simulink model "feedback_harness"  (R2013a)
settings: Solver=ode45  StartTime=0.0  StopTime=8  RelTol=1e-3
settings Model: ModifiedByFormat=The MathWorks Inc.  Creator=The MathWorks Inc.  LastModifiedBy=The MathWorks Inc.
settings DataIOCC: SaveOutput=off  SaveTime=off
settings OptimizationCC: ExpressionDepthLimit=2147483647  LifeSpan=1
settings DebuggingCC: FcnCallInpInsideContextMsg=EnableAllAsWarning
settings GRTTargetCC: CombineOutputUpdateFcns=off  GRTInterface=on

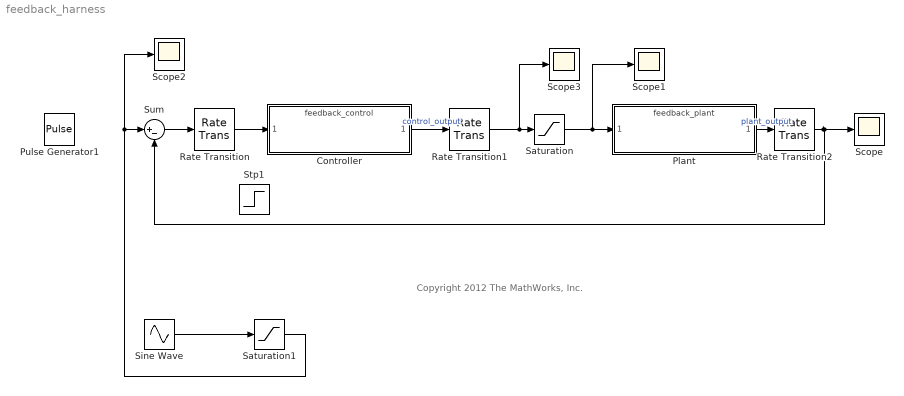
== system feedback_harness ==
  note: Copyright 2012 The MathWorks, Inc.
  Controller : ModelReference  ModelNameDialog=feedback_control  SimulationMode=Normal  ModelReferenceVersion=1.59  CopyOfModelName=feedback_control  DefaultDataLogging=on
  Plant : ModelReference  ModelNameDialog=feedback_plant  SimulationMode=Normal  ModelReferenceVersion=1.26  CopyOfModelName=feedback_plant  DefaultDataLogging=on
  Pulse Generator1 : DiscretePulseGenerator  Period=4000  PulseWidth=2000  SampleTime=0.001
  Rate Transition : RateTransition
  Rate Transition1 : RateTransition  OutPortSampleTime=0.001
  Rate Transition2 : RateTransition
  Saturation : Saturate  UpperLimit=10  LowerLimit=-10
  Saturation1 : Saturate  UpperLimit=1  LowerLimit=-1
  Scope{,1..3} (4 alike) : Scope
      Scope settings: YMin=0  YMax=1.4
      Scope1 settings: YMin=0  YMax=1.4
      Scope2 settings: YMin=0  YMax=1.4  SaveName=ScopeData2
      Scope3 settings: SaveName=ScopeData3
  Sine Wave : Sin  Amplitude=10  Frequency=1.5708  SampleTime=0.001
  Sum : Sum  Inputs=|+-
  Stp1 : Step  IOType=siggen  Time=4  SampleTime=0
  wires:
  Controller/1 -> Rate Transition1/1  "control_output"
  Plant/1 -> Rate Transition2/1  "plant_output"
  Sum/1 -> Rate Transition/1
  Saturation/1 -> Scope1/1, Plant/1
  Sine Wave/1 -> Saturation1/1
  Rate Transition1/1 -> Scope3/1, Saturation/1
  Rate Transition/1 -> Controller/1
  Rate Transition2/1 -> Sum/2, Scope/1
  Saturation1/1 -> Scope2/1, Sum/1
